simulink model "sim10"  (R2015b)
settings: Solver=VariableStepAuto  StartTime=0.0  StopTime=10.0  RelTol=1e-3
values from neighbouring files (symbols this model uses):
  beta = 0.001    [Lab3.m]    (also in calc_erro_l1.m; calc_erro_l2.m)
  dteta_inicial = 0    [Lab3.m]    (also in calc_erro_l1.m; calc_erro_l2.m)
  g = 9.8    [Lab3.m]    (also in calc_erro_l1.m; calc_erro_l2.m)
  k = 0.35    [Lab3.m]    (also in calc_erro_l1.m; calc_erro_l2.m; calc_media_BPM.m = 2)
  L = 0.25    [Lab3.m]    (also in calc_erro_l1.m; calc_erro_l2.m)
  l = 0.2289    [Lab3.m]    (also in calc_erro_l1.m = x; calc_erro_l2.m = x; parametros_estimados.m = l_set(ind_c))
  M = 0.1    [Lab3.m]    (also in calc_erro_l1.m; calc_erro_l2.m)
  m = 0.0799    [Lab3.m]    (also in calc_erro_l1.m; calc_erro_l2.m; parametros_estimados.m = m_set(ind_r))
  T = 0    [Lab3.m]    (also in calc_erro_l1.m; calc_erro_l2.m)
  teta_inicial = pi/4    (= 0.785398163397)    [Lab3.m]    (also in calc_erro_l1.m; calc_erro_l2.m)
settings Model: Creator=Alice  LastModifiedBy=Alice

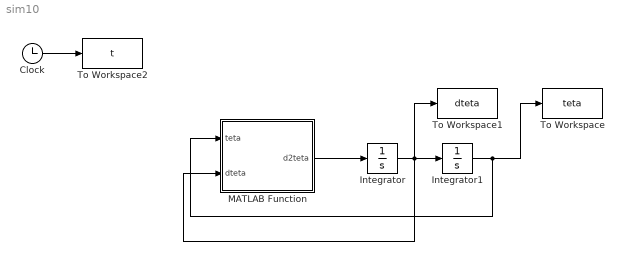
== system sim10 ==
  Clock : Clock
  Integrator : Integrator  InitialCondition=dteta_inicial
  Integrator1 : Integrator  InitialCondition=teta_inicial
  MATLAB Function : MATLAB Function  TreatAsAtomicUnit=on
  To Workspace : ToWorkspace  VariableName=teta  SampleTime=0.01
  To Workspace1 : ToWorkspace  VariableName=dteta  SampleTime=0.01
  To Workspace2 : ToWorkspace  VariableName=t  SampleTime=0.01
  wires:
  MATLAB Function/1(d2teta) -> Integrator/1
  Integrator/1 -> To Workspace1/1, MATLAB Function/2(dteta), Integrator1/1
  Integrator1/1 -> To Workspace/1, MATLAB Function/1(teta)
  Clock/1 -> To Workspace2/1

== matlab function sim10/MATLAB Function ==
  data: teta input; d2teta output; dteta input size=1; T parameter; m parameter; l parameter; M parameter; L parameter; g parameter; k parameter; beta parameter
function d2teta = fcn(teta,dteta, T, m, l, M, L, g, k, beta)
%#codegen
J=(m*l^2)+(M/3)*L^2;
d2teta =(1/J)*(-k*teta*(1+(teta^2/100))-beta*dteta+g*sin(teta)*(m*l+(1/2)*M*L)+T);
